simulink library "elementsLibrary"  (R2018a)
settings: Solver=VariableStepAuto  StartTime=0.0  StopTime=10.0  RelTol=1e-3
undefined symbols (not defined in the file): aerodynamics, ascent, avionics, environment, payload, propulsion, pvessel, recovery, rocket, sequencer
libraries: snippetLibrary x43, $bdroot x24, sharedutil x8, theirs_elementsLibrary x3, simulink_extras x1, aerolibutil x1
(part 2 of 4)

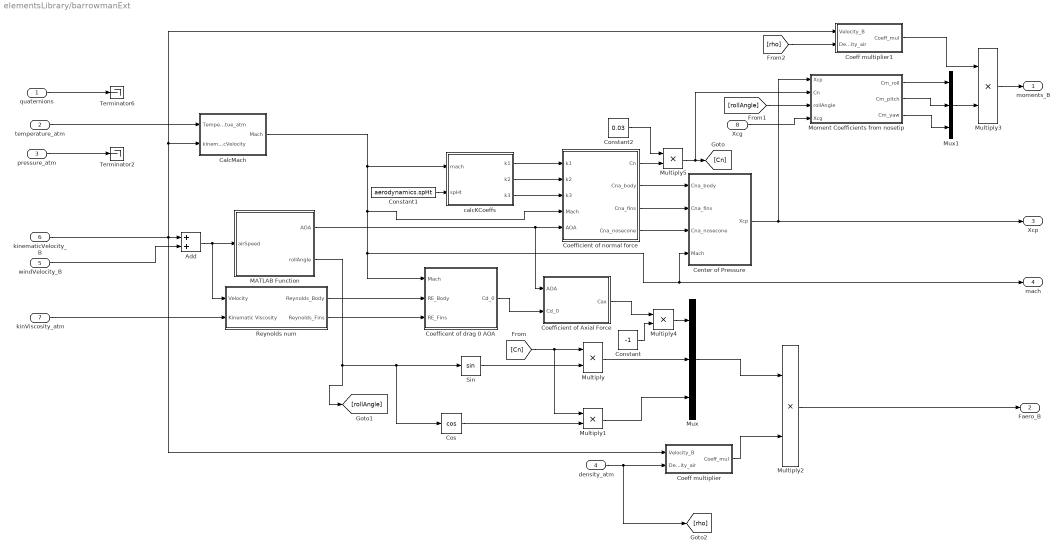
== system elementsLibrary/barrowmanExt ==
  quaternions : Inport
  temperature_atm : Inport  Port=2
  pressure_atm : Inport  Port=3
  density_atm : Inport  Port=4
  windVelocity_B : Inport  Port=5
  kinematicVelocity_B : Inport  Port=6
  kinViscosity_atm : Inport  Port=7
  Xcg : Inport  Port=8
  Add : Sum
  CalcMach : Subsystem
  Center of Pressure : Subsystem
  Coeff multiplier : Subsystem
  Coeff multiplier1 : Subsystem
  Coefficent of drag 0 AOA : Subsystem
  Coefficient of Axial Force : Subsystem
  Coefficient of normal force : Subsystem
  Constant : Constant  Value=-1
  Constant1 : Constant  Value=aerodynamics.spHt
  Constant2 : Constant  Value=0.03
  Cos : Trigonometry  Operator=cos
  MATLAB Function : MATLAB Function  TreatAsAtomicUnit=on
  Moment Coefficients from nosetip : Subsystem
  Multiply{,1..5} (6 alike) : Product
  Mux : Mux  Inputs=3
  Mux1 : Mux  Inputs=3
  Reynolds num : Subsystem
  Sin : Trigonometry
  Terminator2 : Terminator
  Terminator6 : Terminator
  calcKCoeffs : MATLAB Function  TreatAsAtomicUnit=on
  moments_B : Outport
  Faero_B : Outport  Port=2
  Xcp : Outport  Port=3
  mach : Outport  Port=4
  wires:
  pressure_atm/1 -> Terminator2/1
  temperature_atm/1 -> CalcMach/1(Temperatue_atm)
  kinViscosity_atm/1 -> Reynolds num/2(Kinematic Viscosity)
  quaternions/1 -> Terminator6/1
  Add/1 -> Reynolds num/1(Velocity), MATLAB Function/1(airSpeed)
  windVelocity_B/1 -> Add/2
  Reynolds num/1(Reynolds_Body) -> Coefficent of drag 0 AOA/2(RE_Body)
  Reynolds num/2(Reynolds_Fins) -> Coefficent of drag 0 AOA/3(RE_Fins)
  MATLAB Function/1(AOA) -> Coefficient of Axial Force/1(AOA), Coefficient of normal force/5(AOA)
  calcKCoeffs/3(k3) -> Coefficient of normal force/3(k3)
  calcKCoeffs/2(k2) -> Coefficient of normal force/2(k2)
  calcKCoeffs/1(k1) -> Coefficient of normal force/1(k1)
  Constant1/1 -> calcKCoeffs/2(spHt)
  Mux/1 -> Multiply2/1
  CalcMach/1(Mach) -> calcKCoeffs/1(mach), Coefficient of normal force/4(Mach), Coefficent of drag 0 AOA/1(Mach), Center of Pressure/4(Mach), mach/1
  Center of Pressure/1(Xcp) -> Xcp/1, Moment Coefficients from nosetip/1(Xcp)
  Coeff multiplier/1(Coeff_mul) -> Multiply2/2
  Coefficent of drag 0 AOA/1(Cd_0) -> Coefficient of Axial Force/2(Cd_0)
  Coefficient of normal force/2(Cna_body) -> Center of Pressure/1(Cna_body)
  Coefficient of normal force/3(Cna_fins) -> Center of Pressure/2(Cna_fins)
  Coefficient of normal force/4(Cna_nosecone) -> Center of Pressure/3(Cna_nosecone)
  [Cn] -> Multiply/1, Multiply1/1
  Multiply1/1 -> Mux/3
  Multiply2/1 -> Faero_B/1
  Multiply/1 -> Mux/2
  Sin/1 -> Multiply/2
  density_atm/1 -> [rho], Coeff multiplier/2(Density_air)
  kinematicVelocity_B/1 -> Coeff multiplier/1(Velocity_B), Add/1, CalcMach/2(kinematicVelocity), Coeff multiplier1/1(Velocity_B)
  Cos/1 -> Multiply1/2
  MATLAB Function/2(rollAngle) -> [rollAngle], Cos/1, Sin/1
  [rollAngle] -> Moment Coefficients from nosetip/3(rollAngle)
  Moment Coefficients from nosetip/1(Cm_roll) -> Mux1/1
  Moment Coefficients from nosetip/2(Cm_pitch) -> Mux1/2
  Moment Coefficients from nosetip/3(Cm_yaw) -> Mux1/3
  Mux1/1 -> Multiply3/2
  Coeff multiplier1/1(Coeff_mul) -> Multiply3/1
  Multiply3/1 -> moments_B/1
  [rho] -> Coeff multiplier1/2(Density_air)
  Xcg/1 -> Moment Coefficients from nosetip/4(Xcg)
  Multiply4/1 -> Mux/1
  Coefficient of Axial Force/1(Cax) -> Multiply4/1
  Constant/1 -> Multiply4/2
  Coefficient of normal force/1(Cn) -> Multiply5/2
  Multiply5/1 -> Moment Coefficients from nosetip/2(Cn), [Cn]
  Constant2/1 -> Multiply5/1

== system elementsLibrary/environment ==
  altitude_E : Inport
  Earthv1 : $bdroot/Earthv1  environment=environment
  windVelocity_E : Outport
  Temperature : Outport  Port=2
  Pressure : Outport  Port=3
  Density : Outport  Port=4
  kinViscosity_atm : Outport  Port=5
  constants : Outport  Port=6
  wires:
  altitude_E/1 -> Earthv1/1
  Earthv1/1 -> windVelocity_E/1
  Earthv1/2 -> Temperature/1
  Earthv1/3 -> Pressure/1
  Earthv1/4 -> Density/1
  Earthv1/5 -> kinViscosity_atm/1
  Earthv1/6 -> constants/1

== system elementsLibrary/nitrousTank1 ==
  massFlow : Inport
  temperature_atm : Inport  Port=2
  Add : Sum
  Enthalpy of Vapourization : Lookup_n-D  NumberOfTableDimensions=1  BreakpointsForDimension1=pvessel.temperatureBreakpoints  Table=pvessel.delHVap  InternalRulePriority=Speed  RndMeth=Simplest  InputSameDT=on
  Integrator : Integrator
  Integrator1 : Integrator  InitialCondition=pvessel.initOxiTemp
  Nitrous Liq Density : Lookup_n-D  NumberOfTableDimensions=1  BreakpointsForDimension1=pvessel.temperatureBreakpoints  Table=pvessel.liqDensity  InternalRulePriority=Speed  RndMeth=Simplest  InputSameDT=on
  Nitrous Vap Density : Lookup_n-D  NumberOfTableDimensions=1  BreakpointsForDimension1=pvessel.temperatureBreakpoints  Table=pvessel.vapDensity  InternalRulePriority=Speed  RndMeth=Simplest  InputSameDT=on
  Nitrous_Inertia_and_cg : Subsystem
  Saturation Pressures : Lookup_n-D  NumberOfTableDimensions=1  LookupTableObject=SatNitrousTable  BreakpointsForDimension1=pvessel.temperatureBreakpoints  Table=pvessel.pressure  InterpMethod=Linear Lagrange  ExtrapMethod=Clip  DiagnosticForOutOfRangeInput=Warning  InternalRulePriority=Speed  RndMeth=Simplest  InputSameDT=on
  Spec Heat Capacity : Lookup_n-D  NumberOfTableDimensions=1  BreakpointsForDimension1=pvessel.temperatureBreakpoints  Table=pvessel.specHeatCap  InternalRulePriority=Speed  RndMeth=Simplest  InputSameDT=on
  Terminator{,1..3} (4 alike) : Terminator
  Unit Delay : UnitDelay  InitialCondition=pvessel.initLiqMass  SampleTime=-1
  Unit Delay1 : UnitDelay  InitialCondition=pvessel.initOxiTemp  SampleTime=-1
  Unit Delay2 : UnitDelay  InitialCondition=0.001  SampleTime=-1
  Unit Delay3 : UnitDelay  InitialCondition=pvessel.initVapMass  SampleTime=-1
  Unit Delay4 : UnitDelay  InitialCondition=pvessel.initOxiTemp  SampleTime=-1
  Unit Delay5 : UnitDelay  InitialCondition=pvessel.initOxiTemp  SampleTime=-1
  nox_blowdown : MATLAB Function  TreatAsAtomicUnit=on  SystemSampleTime=timeStep  mask{timeStep=pvessel.timeStep, initOxiMass=pvessel.initOxiMass, initLiqMass=pvessel.initLiqMass, tankVolume=pvessel.volumeTank, n2o_pCrit=pvessel.n2o_pCrit, n2o_rhoCrit=pvessel.n2o_rhoCrit, n2o_tCrit=pvessel.n2o_tCrit, n2o_ZCrit=pvessel.n2o_ZCrit, n2o_gamma=pvessel.n2o_gamma}
  output_selection1 : MATLAB Function  TreatAsAtomicUnit=on
  sat_n20_temperature_calc : MATLAB Function  TreatAsAtomicUnit=on
  pressure : Outport
  mass : Outport  Port=2  PortDimensions=1
  rho_oxi : Outport  Port=3
  Oxi_inertia : Outport  Port=4
  X_cg_oxi_engine : Outport  Port=5
  wires:
  output_selection1/1(n2o_sel_p) -> pressure/1, Unit Delay4/1  "pNox"
  massFlow/1 -> Integrator/1
  temperature_atm/1 -> Terminator1/1
  Spec Heat Capacity/1 -> sat_n20_temperature_calc/2(specHtCp)  "specHCapNox"
  Enthalpy of Vapourization/1 -> sat_n20_temperature_calc/3(enthVap)  "enthVapNox"
  Nitrous Liq Density/1 -> output_selection1/4(satLiqDens), nox_blowdown/2(liquidDens)  "satRhoLiqNox"
  Nitrous Vap Density/1 -> nox_blowdown/3(vapDens)  "satRhoVapNox"
  Saturation Pressures/1 -> output_selection1/1(n2o_sat_pressure)
  nox_blowdown/2(liquidMass) -> Unit Delay/1  "liqMassNox"
  Integrator/1 -> nox_blowdown/1(massGone)
  nox_blowdown/4(vapourizedMass) -> Unit Delay2/1  "vapourizedMassNox"
  nox_blowdown/1(vapMass) -> Unit Delay3/1
  Unit Delay2/1 -> sat_n20_temperature_calc/5(vapourizedMass), nox_blowdown/6(oldVapourizedMass)
  Unit Delay/1 -> sat_n20_temperature_calc/4(liquidMass), nox_blowdown/5(oldLiquidMass), output_selection1/2(liquidMass), Add/2  "mass_oxi"
  sat_n20_temperature_calc/1(temperature) -> Unit Delay1/1
  sat_n20_temperature_calc/2(deltaTemp) -> Integrator1/1
  Unit Delay1/1 -> output_selection1/5(satLiqTemp), sat_n20_temperature_calc/1(oldTemperature), Spec Heat Capacity/1, Enthalpy of Vapourization/1, Nitrous Liq Density/1, Saturation Pressures/1, Nitrous Vap Density/1  "SatTemperatureNox"
  Integrator1/1 -> Terminator/1  "inte_delT"
  Unit Delay3/1 -> output_selection1/3(vapMass), Add/1  "vapMassNox"
  output_selection1/2(n2o_sel_rho) -> rho_oxi/1, Nitrous_Inertia_and_cg/2(density)  "rhoNox"
  nox_blowdown/5(vapourDens) -> output_selection1/6(vapDens)
  nox_blowdown/6(vapourTemp) -> output_selection1/7(vapTemp)
  output_selection1/3(n2o_sel_Temp) -> Terminator3/1, Unit Delay5/1  "tempNox"
  nox_blowdown/7(vapourPres) -> output_selection1/8(vapPres)
  Unit Delay4/1 -> nox_blowdown/4(tankPressure)
  Unit Delay5/1 -> nox_blowdown/7(vapTemp)
  Nitrous_Inertia_and_cg/1(Inertia_oxi) -> Oxi_inertia/1
  Nitrous_Inertia_and_cg/2(X_cg) -> X_cg_oxi_engine/1  "X_cg_oxi_engine"
  nox_blowdown/3(massProp) -> Terminator2/1
  Add/1 -> mass/1, Nitrous_Inertia_and_cg/1(mass)

== system elementsLibrary/payload ==
  In1 : Inport
  payload2021 : $bdroot/payload2021  payload=payload
  Out1 : Outport
  wires:
  In1/1 -> payload2021/1
  payload2021/1 -> Out1/1

== system elementsLibrary/payload2021 ==
  Env_temp : Inport
  Input : Inport  Port=2
  Input1 : Inport  Port=3
  Payload_Samples_Temperature : Outport
  Rate_of_Heat_Transfer_Env_Sample : Outport  Port=2
  Payload_Pressure : Outport  Port=3
  Total_Heat_Transfer : Outport  Port=4
  Mass_Dry_Ice : Outport  Port=5

== system elementsLibrary/propulsion ==
  time : Inport
  valveCmd : Inport  Port=2
  temp_atm : Inport  Port=3
  pressure_atm : Inport  Port=4
  "density_atm " : Inport  Port=5
  HREV1 : $bdroot/HREV1  propulsion=propulsion
  gnd{1..4} (4 alike) : Ground
  thrust_B : Outport
  Ve_gas : Outport  Port=2
  propellantMass : Outport  Port=3
  propellantInertias : Outport  Port=4
  engineProperties : Outport  Port=5
  Ve_gas1 : Outport  Port=6
  engineMass : Outport  Port=7
  wires:
  time/1 -> HREV1/1
  valveCmd/1 -> HREV1/2
  temp_atm/1 -> HREV1/3
  pressure_atm/1 -> HREV1/4
  "density_atm "/1 -> HREV1/5
  HREV1/1 -> thrust_B/1
  HREV1/4 -> propellantInertias/1
  HREV1/5 -> engineProperties/1
  HREV1/2 -> Ve_gas1/1
  HREV1/3 -> engineMass/1
  gnd2/1 -> Ve_gas/1
  gnd3/1 -> propellantMass/1

== system elementsLibrary/pvessel ==
  massFlow : Inport
  temperature_atm : Inport  Port=2
  nitrousTank1 : $bdroot/nitrousTank1  pvessel=pvessel
  pressure : Outport
  mass : Outport  Port=2
  rho_oxi : Outport  Port=3
  wires:
  massFlow/1 -> nitrousTank1/1
  temperature_atm/1 -> nitrousTank1/2
  nitrousTank1/1 -> pressure/1
  nitrousTank1/2 -> mass/1
  nitrousTank1/3 -> rho_oxi/1

== system elementsLibrary/recovery ==
  windVelocity : Inport
  density_atm : Inport  Port=2
  envConstants : Inport  Port=3
  inQuaternions : Inport  Port=4
  initVelocity_E : Inport  Port=5
  initPosition_E : Inport  Port=6
  inAngVel : Inport  Port=7
  descentOneDeploy : Inport  Port=8
  descentTwoDeploy : Inport  Port=9
  flightState : Inport  Port=10
  SingleChute : $bdroot/SingleChute  recovery=recovery
  orientationP : Outport
  angularVelocityP : Outport  Port=2
  angularAccelerationP : Outport  Port=3
  angularAccelerationR : Outport  Port=4
  orientationR : Outport  Port=5
  angularVelocityR : Outport  Port=6
  posP_E : Outport  Port=7
  posR_E : Outport  Port=8
  velocityP_E : Outport  Port=9
  velocityR_E : Outport  Port=10
  accelerationR_E : Outport  Port=11
  accelerationP_E : Outport  Port=12
  wires:
  windVelocity/1 -> SingleChute/1
  density_atm/1 -> SingleChute/2
  envConstants/1 -> SingleChute/3
  inQuaternions/1 -> SingleChute/4
  initVelocity_E/1 -> SingleChute/5
  initPosition_E/1 -> SingleChute/6
  inAngVel/1 -> SingleChute/7
  descentOneDeploy/1 -> SingleChute/8
  descentTwoDeploy/1 -> SingleChute/9
  flightState/1 -> SingleChute/10
  SingleChute/1 -> orientationP/1
  SingleChute/2 -> angularVelocityP/1
  SingleChute/3 -> angularAccelerationP/1
  SingleChute/4 -> angularAccelerationR/1
  SingleChute/5 -> orientationR/1
  SingleChute/6 -> angularVelocityR/1
  SingleChute/7 -> posP_E/1
  SingleChute/8 -> posR_E/1
  SingleChute/9 -> velocityP_E/1
  SingleChute/10 -> velocityR_E/1
  SingleChute/11 -> accelerationR_E/1
  SingleChute/12 -> accelerationP_E/1

== system elementsLibrary/rocket ==
  time : Inport
  Jackalope : $bdroot/Jackalope  rocket=rocket
  acceleration_E : Outport
  angularAcceleration_B : Outport  Port=2
  angularVelocity_B : Outport  Port=3
  position_E : Outport  Port=4
  orientation : Outport  Port=5
  velocity_E : Outport  Port=6
  wires:
  time/1 -> Jackalope/1
  Jackalope/1 -> acceleration_E/1
  Jackalope/2 -> angularAcceleration_B/1
  Jackalope/3 -> angularVelocity_B/1
  Jackalope/4 -> position_E/1
  Jackalope/5 -> orientation/1
  Jackalope/6 -> velocity_E/1

== system elementsLibrary/sequencer ==
  position_E : Inport
  orientation : Inport  Port=2
  velocity_E : Inport  Port=3
  thrust_B : Inport  Port=4
  descentOneDeploy : Inport  Port=5
  descentTwoDeploy : Inport  Port=6
  FSv1 : $bdroot/FSv1  sequencer=sequencer
  flightState : Outport
  towerVector : Outport  Port=2
  wires:
  position_E/1 -> FSv1/1
  orientation/1 -> FSv1/2
  velocity_E/1 -> FSv1/3
  thrust_B/1 -> FSv1/4
  descentOneDeploy/1 -> FSv1/5
  descentTwoDeploy/1 -> FSv1/6
  FSv1/1 -> flightState/1
  FSv1/2 -> towerVector/1

== system elementsLibrary/Ascentv1/Calculate Aero Coeffs & Center of Pressure ==
  kinematicVelocity_B : Inport
  temperpature_atm : Inport  Port=2
  pressure_atm : Inport  Port=3
  kinViscosity_atm : Inport  Port=4
  density_atm : Inport  Port=5
  windVelocity_B : Inport  Port=6
  Add1 : Sum
  Terminator{,1..6} (7 alike) : Terminator
  calcAeroCoeffs : MATLAB Function  TreatAsAtomicUnit=on  mask{lw=ascent.aerodynamics.lw, lr=ascent.aerodynamics.lr, lt=ascent.aerodynamics.lt, ls=ascent.aerodynamics.ls, A_fwt=ascent.aerodynamics.A_fwt, Ar=ascent.aerodynamics.Ar, Ap=ascent.aerodynamics.Ap, df=ascent.aerodynamics.df, nf=ascent.aerodynamics.nf, dn=ascent.aerodynamics.dn, du=ascent.aerodynamics.du, ln=ascent.aerodynamics.ln, lb=ascent.aerodynamics.lb, CNalpha_nose=ascent.aerodynamics.CNalpha_nose, Xcp_nose=ascent.aerodynamics.Xcp_nose, Xcp_body=ascent.aerodynamics.Xcp_body, Xcp_fins=ascent.aerodynamics.Xcp_fins, Xf=ascent.aerodynamics.Xf}
  calculate AOA & Side Slip : Subsystem
  calculate Mach : Subsystem
  calculate ZAOA_cd : Subsystem
  Ca_B : Outport
  Cy_B : Outport  Port=2
  Cz_B : Outport  Port=3
  Xcp : Outport  Port=4
  mach : Outport  Port=5
  wires:
  pressure_atm/1 -> Terminator1/1
  temperpature_atm/1 -> calculate Mach/1(temperature_atm)
  kinViscosity_atm/1 -> calculate ZAOA_cd/3(kinViscosity_atm)
  density_atm/1 -> calculate ZAOA_cd/2(density_atm)
  calculate Mach/2(speed of sound) -> Terminator2/1
  calculate Mach/1(mach) -> calcAeroCoeffs/1(mach), mach/1  "mach"
  Add1/1 -> calculate Mach/2(apparentVelocity_E), calculate AOA & Side Slip/1(apparentVelocity_B), calcAeroCoeffs/5(Va), calculate ZAOA_cd/1(apparentVelocity_B)  "Va_B"
  kinematicVelocity_B/1 -> Add1/1
  windVelocity_B/1 -> Add1/2
  calcAeroCoeffs/5(Xcp) -> Xcp/1  "Xcp"
  calcAeroCoeffs/4(Cz_B) -> Cz_B/1  "Cz_B"
  calcAeroCoeffs/3(Cy_B) -> Cy_B/1  "Cy_B"
  calcAeroCoeffs/2(Ca_B) -> Ca_B/1  "Ca_B"
  calcAeroCoeffs/1(Cn_B) -> Terminator/1  "Cn_B"
  calculate ZAOA_cd/1(ZAOA_cd) -> calcAeroCoeffs/2(cd)  "cd"
  calculate AOA & Side Slip/1(AOA) -> calcAeroCoeffs/3(AOA)  "AOA"
  calculate AOA & Side Slip/2(aeroRollAngle) -> calcAeroCoeffs/4(aeroRollAngle)  "aeroRollAngle"
  calcAeroCoeffs/6(Cm_B) -> Terminator3/1  "Cm_B"
  calcAeroCoeffs/7(CN_body) -> Terminator4/1  "CN_body"
  calcAeroCoeffs/8(CN_nose) -> Terminator5/1  "CN_nose"
  calcAeroCoeffs/9(CN_fins) -> Terminator6/1  "CN_fins"

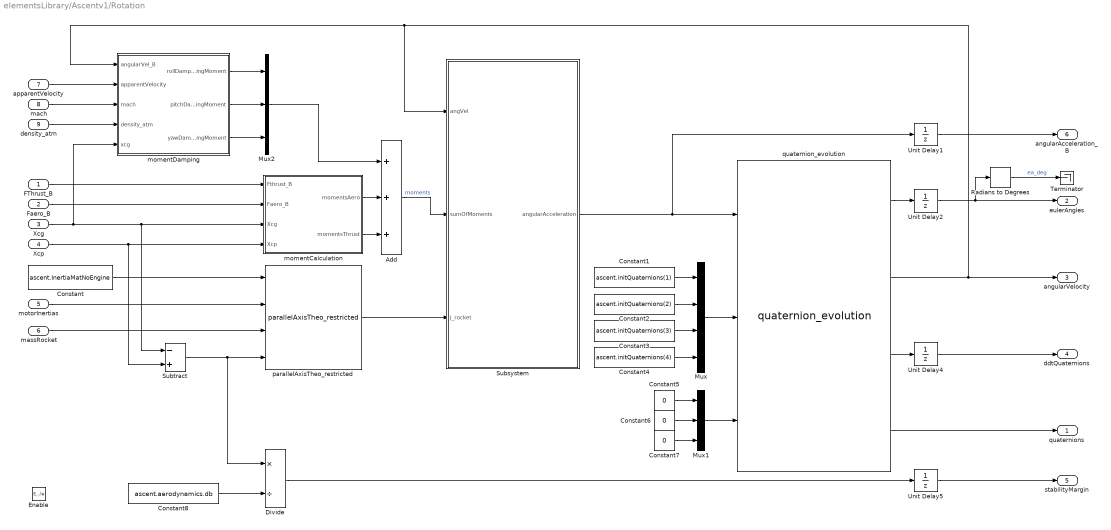
== system elementsLibrary/Ascentv1/Rotation ==
  FThrust_B : Inport
  Faero_B : Inport  Port=2
  Xcg : Inport  Port=3
  Xcp : Inport  Port=4
  motorInertias : Inport  Port=5
  massRocket : Inport  Port=6
  apparentVelocity : Inport  Port=7
  mach : Inport  Port=8
  density_atm : Inport  Port=9
  Enable : EnablePort  StatesWhenEnabling=reset
  Add : Sum  Inputs=3
  Constant : Constant  Value=ascent.InertiaMatNoEngine
  Constant1 : Constant  Value=ascent.initQuaternions(1)
  Constant2 : Constant  Value=ascent.initQuaternions(2)
  Constant3 : Constant  Value=ascent.initQuaternions(3)
  Constant4 : Constant  Value=ascent.initQuaternions(4)
  Constant5 : Constant  Value=0
  Constant6 : Constant  Value=0
  Constant7 : Constant  Value=0
  Constant8 : Constant  Value=ascent.aerodynamics.db
  Divide : Product  Inputs=*/
  Mux : Mux
  Mux1 : Mux  Inputs=3
  Mux2 : Mux  Inputs=3
  Radians to Degrees : simulink_extras/Transformations/Radians to Degrees
  Subsystem : Subsystem
  Subtract : Sum  Inputs=-+
  Terminator : Terminator
  Unit Delay{1..2,4..5} (4 alike) : UnitDelay  SampleTime=-1
  momentCalculation : Subsystem
  momentDamping : Subsystem
  parallelAxisTheo_restricted : snippetLibrary/dynamicsSnippets/parallelAxisTheo_restricted
  quaternion_evolution : snippetLibrary/mathSnippets/quaternion_evolution
  quaternions : Outport
  eulerAngles : Outport  Port=2
  angularVelocity : Outport  Port=3
  ddtQuaternions : Outport  Port=4
  stabilityMargin : Outport  Port=5
  angularAcceleration_B : Outport  Port=6
  wires:
  quaternion_evolution/1 -> Unit Delay2/1
  FThrust_B/1 -> momentCalculation/1(Fthrust_B)
  Faero_B/1 -> momentCalculation/2(Faero_B)
  motorInertias/1 -> parallelAxisTheo_restricted/2
  Constant/1 -> parallelAxisTheo_restricted/1
  massRocket/1 -> parallelAxisTheo_restricted/3
  parallelAxisTheo_restricted/1 -> Subsystem/3(J_rocket)
  quaternion_evolution/3 -> Unit Delay4/1
  Mux/1 -> quaternion_evolution/2
  Constant1/1 -> Mux/1
  Constant2/1 -> Mux/2
  Constant3/1 -> Mux/3
  Constant4/1 -> Mux/4
  Subtract/1 -> parallelAxisTheo_restricted/4, Divide/1
  Xcp/1 -> momentCalculation/4(Xcp), Subtract/2
  Xcg/1 -> momentDamping/5(xcg), momentCalculation/3(Xcg), Subtract/1
  Mux1/1 -> quaternion_evolution/3
  Constant5/1 -> Mux1/1
  Constant6/1 -> Mux1/2
  Constant7/1 -> Mux1/3
  Subsystem/1(angularAcceleration) -> Unit Delay1/1, quaternion_evolution/1
  quaternion_evolution/4 -> quaternions/1
  Unit Delay2/1 -> Radians to Degrees/1, eulerAngles/1
  quaternion_evolution/2 -> angularVelocity/1, Subsystem/1(angVel), momentDamping/1(angularVel_B)
  Unit Delay4/1 -> ddtQuaternions/1
  Unit Delay5/1 -> stabilityMargin/1
  Unit Delay1/1 -> angularAcceleration_B/1
  Radians to Degrees/1 -> Terminator/1  "ea_deg"
  Divide/1 -> Unit Delay5/1
  Constant8/1 -> Divide/2
  mach/1 -> momentDamping/3(mach)
  apparentVelocity/1 -> momentDamping/2(apparentVelocity)
  momentDamping/1(rollDampingMoment) -> Mux2/1
  momentDamping/2(pitchDampingMoment) -> Mux2/2
  momentDamping/3(yawDampingMoment) -> Mux2/3
  Mux2/1 -> Add/1
  momentCalculation/1(momentsAero) -> Add/2
  momentCalculation/2(momentsThrust) -> Add/3
  Add/1 -> Subsystem/2(sumOfMoments)  "moments"
  density_atm/1 -> momentDamping/4(density_atm)

== system elementsLibrary/Ascentv1/Tower_Correction ==
  flightState : Inport
  quaternionsIn : Inport  Port=2
  eulerAnglesIn : Inport  Port=3
  angularVelocityIn : Inport  Port=4
  ddtQuaternionsIn : Inport  Port=5
  stabilityMarginIn : Inport  Port=6
  angularAccelerationIn_B : Inport  Port=7
  Constant : Constant
  Constant1 : Constant  Value=ascent.initQuaternions(1)
  Constant{5..11} (7 alike) : Constant  Value=0
  Constant2 : Constant  Value=ascent.initQuaternions(2)
  Constant3 : Constant  Value=ascent.initQuaternions(3)
  Constant4 : Constant  Value=ascent.initQuaternions(4)
  Mux : Mux
  Mux1 : Mux  Inputs=3
  Mux2 : Mux
  NotEqual : RelationalOperator  Operator=~=  OutDataTypeStr=boolean  RndMeth=Simplest
  Switch{,2..3,5} (4 alike) : Switch  Criteria=u2 ~= 0
  quaternions : Outport
  eulerAngles : Outport  Port=2
  angularVelocity : Outport  Port=3
  ddtQuaternions : Outport  Port=4
  stabilityMargin : Outport  Port=5
  angularAcceleration_B : Outport  Port=6
  wires:
  quaternionsIn/1 -> Switch/1
  Switch/1 -> quaternions/1
  angularVelocityIn/1 -> Switch2/1
  ddtQuaternionsIn/1 -> Switch3/1
  angularAccelerationIn_B/1 -> Switch5/1
  eulerAnglesIn/1 -> eulerAngles/1
  Switch2/1 -> angularVelocity/1
  Switch3/1 -> ddtQuaternions/1
  stabilityMarginIn/1 -> stabilityMargin/1
  Switch5/1 -> angularAcceleration_B/1
  flightState/1 -> NotEqual/1
  Constant/1 -> NotEqual/2
  NotEqual/1 -> Switch3/2, Switch5/2, Switch2/2, Switch/2
  Constant1/1 -> Mux/1
  Constant2/1 -> Mux/2
  Constant3/1 -> Mux/3
  Constant5/1 -> Mux1/1
  Constant6/1 -> Mux1/2
  Mux/1 -> Switch/3
  Constant7/1 -> Mux1/3
  Constant4/1 -> Mux/4
  Mux1/1 -> Switch2/3, Switch5/3
  Constant10/1 -> Mux2/3
  Constant8/1 -> Mux2/1
  Constant9/1 -> Mux2/2
  Mux2/1 -> Switch3/3
  Constant11/1 -> Mux2/4

== system elementsLibrary/Ascentv1/Translation ==
  Faero_E : Inport
  FThrust_E : Inport  Port=2
  Fg_E : Inport  Port=3
  massRocket : Inport  Port=4
  Enable : EnablePort  StatesWhenEnabling=reset
  Add : Sum  Inputs=+++
  Divide : Product  Inputs=*/
  Integrator : Integrator
  Integrator1 : Integrator  InitialCondition=[0;0;ascent.aerodynamics.l_TR/2]
  position_E : Outport
  velocity_E : Outport  Port=2
  acceleration_E : Outport  Port=3
  wires:
  Fg_E/1 -> Add/3
  Faero_E/1 -> Add/1
  FThrust_E/1 -> Add/2
  Add/1 -> Divide/1
  massRocket/1 -> Divide/2
  Divide/1 -> acceleration_E/1, Integrator/1  "acceleration_E"
  Integrator/1 -> velocity_E/1, Integrator1/1  "velocity_E"
  Integrator1/1 -> position_E/1  "position_E"

== system elementsLibrary/Ascentv1/center of mass//gravity calculation ==
  motorMass : Inport
  motorProperties : Inport  Port=2
  rocketEmptyMass : Inport  Port=3
  rocketEmptyXcg : Inport  Port=4
  Add : Sum
  Add1 : Sum
  Add2 : Sum
  Bus Selector : BusSelector  OutputSignals=x_gm_B,x_cg_B
  Divide : Product  Inputs=*/
  Multiply : Product
  Multiply1 : Product
  Xcg : Outport
  massR : Outport  Port=2
  wires:
  motorProperties/1 -> Bus Selector/1
  Bus Selector/2 -> Add/2  "<x_cg_B>"
  Bus Selector/1 -> Add/1  "<x_gm_B>"
  motorMass/1 -> Multiply/1, Add2/1
  Add/1 -> Multiply/2
  Multiply/1 -> Add1/2
  rocketEmptyMass/1 -> Multiply1/2, Add2/2
  rocketEmptyXcg/1 -> Multiply1/1
  Divide/1 -> Xcg/1
  Add2/1 -> massR/1, Divide/2
  Add1/1 -> Divide/1
  Multiply1/1 -> Add1/1

== system elementsLibrary/Ascentv2/Calculating Mass and XCG ==
  rocketEmptyXcg : Inport
  rocketEmptyMass : Inport  Port=2
  propellantMass : Inport  Port=3
  motorProperties : Inport  Port=4
  Add : Sum
  Add1 : Sum
  Add2 : Sum
  Bus Selector : BusSelector  OutputSignals=x_gm_B,x_cg_B
  Divide : Product  Inputs=*/
  Multiply : Product
  Multiply1 : Product
  massRocket : Outport
  Xcg : Outport  Port=2
  wires:
  Bus Selector/2 -> Add/2  "<x_cg_B>"
  Add2/1 -> massRocket/1, Divide/2
  Divide/1 -> Xcg/1
  rocketEmptyMass/1 -> Multiply1/2, Add2/1
  Add/1 -> Multiply/2
  propellantMass/1 -> Add2/2, Multiply/1
  Bus Selector/1 -> Add/1  "<x_gm_B>"
  Multiply1/1 -> Add1/1
  Add1/1 -> Divide/1
  Multiply/1 -> Add1/2
  rocketEmptyXcg/1 -> Multiply1/1
  motorProperties/1 -> Bus Selector/1

== system elementsLibrary/Ascentv2/Force of Gravity ==
  G_Const : Inport
  massEarth : Inport  Port=2
  radiusEarth : Inport  Port=3
  massRocket : Inport  Port=4
  Altitude : Inport  Port=5
  Add : Sum
  Divide : Product  Inputs=*/
  Gain : Gain  Gain=-1
  Multiply : Product  Inputs=3
  Square : Math  Operator=square  SaturateOnIntegerOverflow=on
  Fg_E : Outport
  wires:
  massRocket/1 -> Multiply/3
  radiusEarth/1 -> Add/1
  Divide/1 -> Fg_E/1
  Altitude/1 -> Add/2
  Add/1 -> Square/1
  Square/1 -> Divide/2
  G_Const/1 -> Multiply/1
  massEarth/1 -> Multiply/2
  Multiply/1 -> Gain/1
  Gain/1 -> Divide/1

== system elementsLibrary/Ascentv2/Forces Body Frame to Earth Frame ==
  Transformation_Matrix : Inport
  F_Aero_B : Inport  Port=2
  F_Thrust_B : Inport  Port=3
  Matrix Multiply : Product  Multiplication=Matrix(*)
  Matrix Multiply1 : Product  Multiplication=Matrix(*)
  F_Aero_E : Outport
  F_Thrust_E : Outport  Port=2
  wires:
  Transformation_Matrix/1 -> Matrix Multiply1/1, Matrix Multiply/1
  F_Aero_B/1 -> Matrix Multiply1/2
  F_Thrust_B/1 -> Matrix Multiply/2
  Matrix Multiply1/1 -> F_Aero_E/1
  Matrix Multiply/1 -> F_Thrust_E/1

== system elementsLibrary/Ascentv2/Rotational ==
  moments_B : Inport
  propellentInertias : Inport  Port=2
  propellantMass : Inport  Port=3
  motorProperties : Inport  Port=4
  rocketEmptyXcg : Inport  Port=5
  Constant1 : Constant  Value=ascent.initQuaternions(1)
  Constant2 : Constant  Value=ascent.initQuaternions(2)
  Constant3 : Constant  Value=ascent.initQuaternions(3)
  Constant4 : Constant  Value=ascent.initQuaternions(4)
  Constant5 : Constant  Value=0.000001
  Constant6 : Constant  Value=0.000001
  Constant7 : Constant  Value=0.000001
  "Inertia_Matrix " : Subsystem
  Mux : Mux
  Mux1 : Mux  Inputs=3
  Subsystem : Subsystem
  Unit Delay{,1..3} (4 alike) : UnitDelay  SampleTime=-1
  quaternion_evolution : Subsystem
  quaternions : Outport
  ddtQuaternions : Outport  Port=2
  eulerAngles : Outport  Port=3
  angularVelocity : Outport  Port=4
  angularAcceleration_B : Outport  Port=5
  wires:
  quaternion_evolution/2(anguarVelocity) -> Unit Delay3/1, angularVelocity/1
  quaternion_evolution/4(quaternions) -> quaternions/1
  Mux/1 -> quaternion_evolution/2(initialQuaternions)
  Constant2/1 -> Mux/2
  Constant5/1 -> Mux1/1
  Constant3/1 -> Mux/3
  Constant6/1 -> Mux1/2
  Constant1/1 -> Mux/1
  Constant7/1 -> Mux1/3
  Constant4/1 -> Mux/4
  Mux1/1 -> quaternion_evolution/3(initialAngVel)
  moments_B/1 -> Subsystem/3(sumOfMoments)
  "Inertia_Matrix "/1(J_rocket) -> Subsystem/2(J_rocket)  "J equivelant"
  propellentInertias/1 -> "Inertia_Matrix "/1(motorInertias)
  propellantMass/1 -> "Inertia_Matrix "/2(propellantMass)
  motorProperties/1 -> "Inertia_Matrix "/3(motorProperties)
  rocketEmptyXcg/1 -> "Inertia_Matrix "/4(rocketEmptyXcg)
  quaternion_evolution/3(ddtQuaternions) -> Unit Delay/1
  Unit Delay/1 -> ddtQuaternions/1
  Unit Delay1/1 -> eulerAngles/1
  quaternion_evolution/1(euler_angles) -> Unit Delay1/1
  Subsystem/1(angularAcceleration) -> Unit Delay2/1
  Unit Delay2/1 -> angularAcceleration_B/1, quaternion_evolution/1(angularAccelerations_B)
  Unit Delay3/1 -> Subsystem/1(angVel)

== system elementsLibrary/Ascentv2/Tower_Correction ==
  flightState : Inport
  quaternionsIn : Inport  Port=2
  ddtQuaternionsIn : Inport  Port=3
  eulerAnglesIn : Inport  Port=4
  angularVelocityIn : Inport  Port=5
  stabilityMarginIn : Inport  Port=6
  angularAccelerationIn_B : Inport  Port=7
  Constant : Constant
  Constant1 : Constant  Value=ascent.initQuaternions(1)
  Constant{5..11} (7 alike) : Constant  Value=0
  Constant2 : Constant  Value=ascent.initQuaternions(2)
  Constant3 : Constant  Value=ascent.initQuaternions(3)
  Constant4 : Constant  Value=ascent.initQuaternions(4)
  Mux : Mux
  Mux1 : Mux  Inputs=3
  Mux2 : Mux
  NotEqual : RelationalOperator  Operator=~=  OutDataTypeStr=boolean  RndMeth=Simplest
  Switch{,2..3,5} (4 alike) : Switch  Criteria=u2 ~= 0
  quaternions : Outport
  eulerAngles : Outport  Port=2
  angularVelocity : Outport  Port=3
  ddtQuaternions : Outport  Port=4
  stabilityMargin : Outport  Port=5
  angularAcceleration_B : Outport  Port=6
  wires:
  quaternionsIn/1 -> Switch/1
  Switch/1 -> quaternions/1
  angularVelocityIn/1 -> Switch2/1
  ddtQuaternionsIn/1 -> Switch3/1
  angularAccelerationIn_B/1 -> Switch5/1
  eulerAnglesIn/1 -> eulerAngles/1
  Switch2/1 -> angularVelocity/1
  Switch3/1 -> ddtQuaternions/1
  stabilityMarginIn/1 -> stabilityMargin/1
  Switch5/1 -> angularAcceleration_B/1
  flightState/1 -> NotEqual/1
  Constant/1 -> NotEqual/2
  NotEqual/1 -> Switch3/2, Switch5/2, Switch2/2, Switch/2
  Constant1/1 -> Mux/1
  Constant2/1 -> Mux/2
  Constant3/1 -> Mux/3
  Constant5/1 -> Mux1/1
  Constant6/1 -> Mux1/2
  Mux/1 -> Switch/3
  Constant7/1 -> Mux1/3
  Constant4/1 -> Mux/4
  Mux1/1 -> Switch2/3, Switch5/3
  Constant10/1 -> Mux2/3
  Constant8/1 -> Mux2/1
  Constant9/1 -> Mux2/2
  Mux2/1 -> Switch3/3
  Constant11/1 -> Mux2/4

== system elementsLibrary/Ascentv2/Translational  ==
  F_Aero_E : Inport
  F_Thrust_E : Inport  Port=2
  Fg_E : Inport  Port=3
  massRocket : Inport  Port=4
  Add : Sum  Inputs=+++
  Divide : Product  Inputs=*/
  Integrator : Integrator
  Integrator1 : Integrator
  Acceleration_E : Outport
  Velocity_E : Outport  Port=2
  Position_E : Outport  Port=3
  wires:
  Integrator1/1 -> Position_E/1
  Divide/1 -> Integrator/1, Acceleration_E/1
  F_Aero_E/1 -> Add/1
  massRocket/1 -> Divide/2
  Integrator/1 -> Velocity_E/1, Integrator1/1
  F_Thrust_E/1 -> Add/2
  Fg_E/1 -> Add/3
  Add/1 -> Divide/1

== system elementsLibrary/Ascentv2/aerodynamics ==
  quaternions : Inport
  airbrakecmd : Inport  Port=2
  temperature_atm : Inport  Port=3
  pressure_atm : Inport  Port=4
  density_atm : Inport  Port=5
  windVelocity_E : Inport  Port=6
  kinematicVelocity_E : Inport  Port=7
  kinViscosity_atm : Inport  Port=8
  Xcg : Inport  Port=9
  Transformation_Matrix : Inport  Port=10
  Invert 3x3 Matrix : aerolibutil/Invert  3x3 Matrix
  Matrix Multiply : Product  Multiplication=Matrix(*)
  Matrix Multiply1 : Product  Multiplication=Matrix(*)
  Terminator1 : Terminator
  barrowmanExt : $bdroot/barrowmanExt  aerodynamics=aerodynamics
  moments_B : Outport
  Faero_B : Outport  Port=2
  Xcp : Outport  Port=3
  mach : Outport  Port=4
  wires:
  barrowmanExt/2 -> Faero_B/1
  pressure_atm/1 -> barrowmanExt/3
  airbrakecmd/1 -> Terminator1/1
  windVelocity_E/1 -> Matrix Multiply/2
  kinematicVelocity_E/1 -> Matrix Multiply1/2
  kinViscosity_atm/1 -> barrowmanExt/7
  density_atm/1 -> barrowmanExt/4
  temperature_atm/1 -> barrowmanExt/2
  quaternions/1 -> barrowmanExt/1
  barrowmanExt/1 -> moments_B/1
  barrowmanExt/3 -> Xcp/1
  barrowmanExt/4 -> mach/1
  Xcg/1 -> barrowmanExt/8
  Transformation_Matrix/1 -> Invert 3x3 Matrix/1
  Invert 3x3 Matrix/1 -> Matrix Multiply1/1, Matrix Multiply/1
  Matrix Multiply1/1 -> barrowmanExt/6
  Matrix Multiply/1 -> barrowmanExt/5

== system elementsLibrary/Earthv1/Wind Velocity Calculation ==
  In1 : Inport
  Altitude : Inport  Port=2
  Atmospheric coefficient : Constant  Value=environment.atmospheric_coeff
  Divide : Product  Inputs=*/
  Height at ground : Constant  Value=environment.referenceWindAltitude
  Multiply : Product
  Power : Math  Operator=pow  SaturateOnIntegerOverflow=on
  Wind Velocity at Ground : Constant  Value=environment.referenceWindSpeed
  Out1 : Outport
  wires:
  Height at ground/1 -> Divide/2
  In1/1 -> Divide/1
  Divide/1 -> Power/1
  Power/1 -> Multiply/1
  Wind Velocity at Ground/1 -> Multiply/2
  Atmospheric coefficient/1 -> Power/2
  Multiply/1 -> Out1/1

== system elementsLibrary/Earthv2/Gravitational Acceleration ==
  Altitude : Inport
  Earth Radius : Inport  Port=2
  Add : Sum
  Constant1 : Constant  Value=environment.MASS_EARTH
  Constant3 : Constant  Value=environment.GRAVITATION_CONST
  Divide : Product  Inputs=*/
  Gain : Gain  Gain=-1
  Multiply : Product
  Square : Math  Operator=square  SaturateOnIntegerOverflow=on
  Acceleration : Outport
  wires:
  Gain/1 -> Acceleration/1
  Divide/1 -> Gain/1
  Multiply/1 -> Divide/1
  Constant3/1 -> Multiply/2
  Constant1/1 -> Multiply/1
  Square/1 -> Divide/2
  Add/1 -> Square/1
  Earth Radius/1 -> Add/2
  Altitude/1 -> Add/1

== system elementsLibrary/Earthv2/Subsystem ==
  Latitude : Inport
  Add : Sum
  Cos1 : Trigonometry  Operator=cos
  Major Radius : Constant  Value=environment.MAJOR_RADIUS_EARTH
  Minor Radius : Constant  Value=environment.MINOR_RADIUS_EARTH
  Multiply2 : Product
  Multiply3 : Product
  Sin1 : Trigonometry
  Sqrt : Sqrt  SaturateOnIntegerOverflow=on
  Square : Math  Operator=square  SaturateOnIntegerOverflow=on
  Square1 : Math  Operator=square  SaturateOnIntegerOverflow=on
  Radius : Outport
  wires:
  Sqrt/1 -> Radius/1
  Minor Radius/1 -> Multiply2/1
  Sin1/1 -> Multiply3/2
  Major Radius/1 -> Multiply3/1
  Multiply2/1 -> Square/1
  Add/1 -> Sqrt/1
  Multiply3/1 -> Square1/1
  Cos1/1 -> Multiply2/2
  Square1/1 -> Add/2
  Square/1 -> Add/1
  Latitude/1 -> Cos1/1, Sin1/1

== system elementsLibrary/Earthv2/Wind Velocity Calculation ==
  Altitude : Inport
  Ground Wind Speed : Inport  Port=2
  Atmospheric coefficient : Constant  Value=environment.atmospheric_coeff
  Divide : Product  Inputs=*/
  Height at ground : Constant  Value=environment.referenceWindAltitude
  Multiply : Product
  Power : Math  Operator=pow  SaturateOnIntegerOverflow=on
  Out1 : Outport
  wires:
  Ground Wind Speed/1 -> Multiply/2
  Multiply/1 -> Out1/1
  Atmospheric coefficient/1 -> Power/2
  Power/1 -> Multiply/1
  Divide/1 -> Power/1
  Altitude/1 -> Divide/1
  Height at ground/1 -> Divide/2

== system elementsLibrary/HREV1/Chamber_Ballistics ==
  mdot_oxi : Inport
  cStar : Inport  Port=2
  Add : Sum
  Constant : Constant  Value=2
  Divide : Product  Inputs=*/
  Grain_outer_dia : Constant  Value=propulsion.Dfg_outer
  Inertia : Subsystem
  Integrator : Integrator  InitialCondition=propulsion.Dfg_inner
  Unit Delay : UnitDelay  SampleTime=-1
  X_grain_length : Constant  Value=propulsion.Lfg
  calc_chamber_params : Subsystem
  calc_mdot_fuel : Subsystem
  calc_port_diameter : Subsystem
  mdot_fuel : Outport
  mdot_total : Outport  Port=2
  Pc : Outport  Port=3
  Tc : Outport  Port=4
  rdot_fuel : Outport  Port=5
  massFlux_oxi : Outport  Port=6
  OF_ratio : Outport  Port=7
  mass_fuel : Outport  Port=8
  Fuel_inertia : Outport  Port=9
  X_cg_fuel : Outport  Port=10
  wires:
  mdot_oxi/1 -> Add/2, calc_port_diameter/1(mdot_oxi), calc_mdot_fuel/1(mdot_oxi)
  calc_port_diameter/1(dDp_dt) -> Integrator/1
  Integrator/1 -> calc_port_diameter/2(Dp_prev), calc_mdot_fuel/2(Dp), Inertia/2(Grain_inner_dia)  "D_port"
  calc_mdot_fuel/1(Gox) -> massFlux_oxi/1
  Add/1 -> mdot_total/1, calc_chamber_params/2(mdot_prop)
  calc_mdot_fuel/3(mdot_f) -> Add/1, mdot_fuel/1
  calc_mdot_fuel/2(rdot_f) -> Unit Delay/1, rdot_fuel/1
  calc_mdot_fuel/4(OF_ratio) -> calc_chamber_params/1(OF_ratio), OF_ratio/1
  calc_chamber_params/2(Tc) -> Tc/1
  calc_chamber_params/1(Pc) -> Pc/1
  cStar/1 -> calc_chamber_params/3(cStar)
  Unit Delay/1 -> calc_port_diameter/3(rdot_f)
  calc_mdot_fuel/5(massFuel) -> mass_fuel/1, Inertia/1(massFuel)
  Grain_outer_dia/1 -> Inertia/3(Grain_outer_dia)
  X_grain_length/1 -> Divide/1, Inertia/4(X_fuel_length)
  Inertia/1(Fuel_inertia) -> Fuel_inertia/1
  Constant/1 -> Divide/2
  Divide/1 -> X_cg_fuel/1

== system elementsLibrary/HREV1/Injecter ==
  "Tank_pressure " : Inport
  Chamber_pressure : Inport  Port=2
  density_oxi : Inport  Port=3
  mass_oxi : Inport  Port=4
  Area_of_injector_hole : Constant  Value=propulsion.A_ih
  Constant : Constant  Value=2
  Constant1 : Constant  Value=0
  GreaterThan : RelationalOperator  Operator=>  OutDataTypeStr=boolean  RndMeth=Simplest
  Injector_discharge_coefficient : Constant  Value=propulsion.injector_Cd
  Kpa_to_Pa : Gain  Gain=1000
  Less Than : RelationalOperator  OutDataTypeStr=boolean  RndMeth=Simplest
  Multiply : Product  Inputs=3
  Multiply1 : Product  Inputs=3
  Multiply2 : Product
  Multiply3 : Product
  Number_of_injector_holes : Constant  Value=propulsion.nIHoles
  Product : Product
  Saturation : Saturate  UpperLimit=10  LowerLimit=0
  Sqrt : Sqrt  SaturateOnIntegerOverflow=on
  Subtract : Sum  Inputs=+-
  mdot_oxi : Outport
  wires:
  Sqrt/1 -> Product/2
  density_oxi/1 -> Multiply1/2
  Constant/1 -> Multiply1/1
  Multiply/1 -> Product/1
  "Tank_pressure "/1 -> Less Than/1, Subtract/1
  Multiply1/1 -> Multiply2/1
  Area_of_injector_hole/1 -> Multiply/2
  Number_of_injector_holes/1 -> Multiply/3
  Product/1 -> Multiply3/1
  Injector_discharge_coefficient/1 -> Multiply/1
  Chamber_pressure/1 -> Less Than/2, Subtract/2
  Subtract/1 -> Kpa_to_Pa/1
  Saturation/1 -> mdot_oxi/1
  Kpa_to_Pa/1 -> Multiply1/3
  Less Than/1 -> Multiply2/2
  Multiply2/1 -> Sqrt/1
  mass_oxi/1 -> GreaterThan/1
  Constant1/1 -> GreaterThan/2
  GreaterThan/1 -> Multiply3/2
  Multiply3/1 -> Saturation/1

== system elementsLibrary/HREV1/Nozzle ==
  mdot : Inport
  Pc : Inport  Port=2
  Tc : Inport  Port=3
  P_atm : Inport  Port=4
  Constant : Constant  Value=0
  Divide : Product  Inputs=*/
  Mux : Mux  Inputs=3
  calc_Vexit : Subsystem
  calc_charVel : Subsystem
  calc_speedOfSound : Subsystem
  calc_thrust : Subsystem
  thrust_B : Outport
  V_exit : Outport  Port=2
  mach_exit : Outport  Port=3
  charV : Outport  Port=4
  wires:
  calc_charVel/1(cStar) -> charV/1
  calc_speedOfSound/1("speedOfSound ") -> Divide/2, calc_charVel/1(speedOfSound)
  Tc/1 -> calc_speedOfSound/1(Tc), calc_Vexit/1(Tc)
  calc_Vexit/1(Ve_gas) -> calc_thrust/2(Ve_gas), Divide/1, V_exit/1
  Divide/1 -> mach_exit/1
  Mux/1 -> thrust_B/1
  Constant/1 -> Mux/2, Mux/3
  P_atm/1 -> calc_thrust/4(Patm), calc_thrust/3(Pe), calc_Vexit/3(Pe)
  Pc/1 -> calc_Vexit/2(Pc)
  calc_thrust/1(axialThrust) -> Mux/1
  mdot/1 -> calc_thrust/1(mdot_prop)

== system elementsLibrary/HREV1/Propellant_Mass ==
  mass_oxi : Inport
  mass_fuel : Inport  Port=2
  Add1 : Sum
  massProp : Outport
  wires:
  Add1/1 -> massProp/1
  mass_oxi/1 -> Add1/1
  mass_fuel/1 -> Add1/2

== system elementsLibrary/HREV1/cg_propellent_engine ==
  X_cg_fuel_engine : Inport
  mass_fuel : Inport  Port=2
  X_cg_oxi_engine : Inport  Port=3
  mass_oxi : Inport  Port=4
  Add : Sum
  Add1 : Sum
  Divide : Product  Inputs=*/
  Multiply : Product
  Multiply1 : Product
  cg_prop_engine : Outport
  wires:
  mass_fuel/1 -> Add1/1, Multiply/2
  X_cg_fuel_engine/1 -> Multiply/1
  X_cg_oxi_engine/1 -> Multiply1/1
  mass_oxi/1 -> Add1/2, Multiply1/2
  Multiply/1 -> Add/1
  Multiply1/1 -> Add/2
  Add/1 -> Divide/1
  Add1/1 -> Divide/2
  Divide/1 -> cg_prop_engine/1

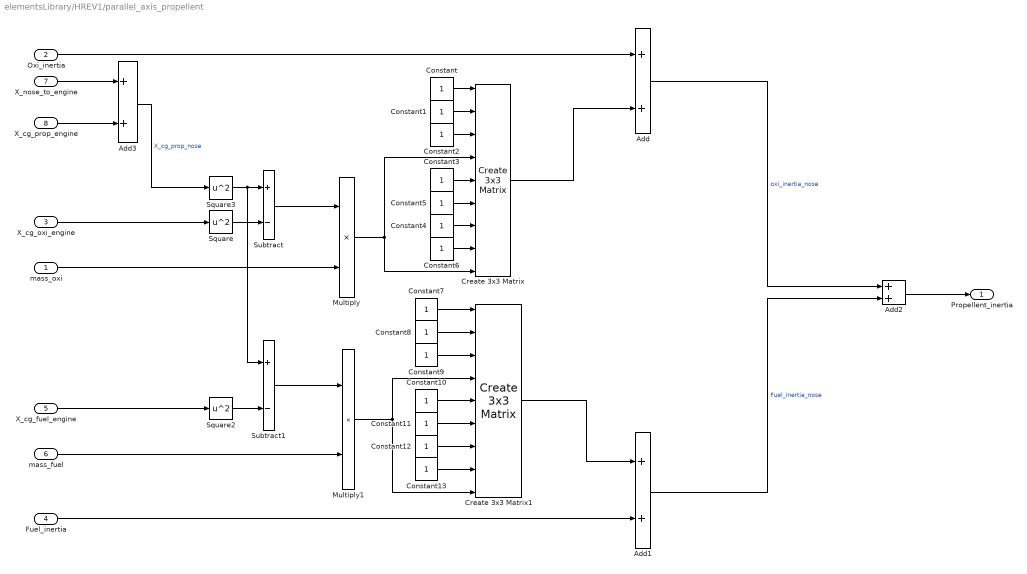
== system elementsLibrary/HREV1/parallel_axis_propellent ==
  mass_oxi : Inport
  Oxi_inertia : Inport  Port=2
  X_cg_oxi_engine : Inport  Port=3
  Fuel_inertia : Inport  Port=4
  X_cg_fuel_engine : Inport  Port=5
  mass_fuel : Inport  Port=6
  X_nose_to_engine : Inport  Port=7
  X_cg_prop_engine : Inport  Port=8
  Add{,1..3} (4 alike) : Sum
  Constant{,1..13} (14 alike) : Constant
  Create 3x3 Matrix : sharedutil/Create 3x3 Matrix  aMode=aMode
  Create 3x3 Matrix1 : sharedutil/Create 3x3 Matrix  aMode=aMode
  Multiply : Product
  Multiply1 : Product
  Square : Math  Operator=square  SaturateOnIntegerOverflow=on
  Square2 : Math  Operator=square  SaturateOnIntegerOverflow=on
  Square3 : Math  Operator=square  SaturateOnIntegerOverflow=on
  Subtract : Sum  Inputs=+-
  Subtract1 : Sum  Inputs=+-
  Propellent_inertia : Outport
  wires:
  X_cg_oxi_engine/1 -> Square/1
  Square3/1 -> Subtract1/1, Subtract/1
  Square/1 -> Subtract/2
  mass_oxi/1 -> Multiply/2
  Subtract/1 -> Multiply/1
  Oxi_inertia/1 -> Add/1
  X_cg_fuel_engine/1 -> Square2/1
  Square2/1 -> Subtract1/2
  Subtract1/1 -> Multiply1/1
  mass_fuel/1 -> Multiply1/2
  Fuel_inertia/1 -> Add1/2
  Constant1/1 -> Create 3x3 Matrix/2
  Constant/1 -> Create 3x3 Matrix/1
  Constant3/1 -> Create 3x3 Matrix/5
  Constant5/1 -> Create 3x3 Matrix/6
  Constant7/1 -> Create 3x3 Matrix1/1
  Constant8/1 -> Create 3x3 Matrix1/2
  Constant9/1 -> Create 3x3 Matrix1/3
  Constant10/1 -> Create 3x3 Matrix1/5
  Constant11/1 -> Create 3x3 Matrix1/6
  Constant12/1 -> Create 3x3 Matrix1/7
  Constant13/1 -> Create 3x3 Matrix1/8
  Constant2/1 -> Create 3x3 Matrix/3
  Add2/1 -> Propellent_inertia/1
  Multiply1/1 -> Create 3x3 Matrix1/4, Create 3x3 Matrix1/9
  Create 3x3 Matrix1/1 -> Add1/1
  Multiply/1 -> Create 3x3 Matrix/4, Create 3x3 Matrix/9
  Constant6/1 -> Create 3x3 Matrix/8
  Constant4/1 -> Create 3x3 Matrix/7
  Create 3x3 Matrix/1 -> Add/2
  Add/1 -> Add2/1  "oxi_inertia_nose"
  Add1/1 -> Add2/2  "Fuel_inertia_nose"
  X_nose_to_engine/1 -> Add3/1
  X_cg_prop_engine/1 -> Add3/2
  Add3/1 -> Square3/1  "X_cg_prop_nose"

== system elementsLibrary/Jackalope/ascent ==
  windVelocity_E : Inport
  temperature_atm : Inport  Port=2
  pressure_atm : Inport  Port=3
  density_atm : Inport  Port=4
  thrust_B : Inport  Port=5
  motorMass : Inport  Port=6
  motorProperties : Inport  Port=7
  envConstants : Inport  Port=8
  flightState : Inport  Port=9
  towerVector : Inport  Port=10
  rocketEmptyMass : Inport  Port=11
  rocketEmptyXcg : Inport  Port=12
  motorInertias : Inport  Port=13
  kinViscosity_atm : Inport  Port=14
  airbrakeCmdAngle : Inport  Port=15
  propellantMass : Inport  Port=16
  propellantInertias : Inport  Port=17
  Ascentv1 : $bdroot/Ascentv1  ascent=ascent
  term16 : Terminator
  term17 : Terminator
  position_E : Outport
  velocity_E : Outport  Port=2
  acceleration_E : Outport  Port=3
  eulerAngles : Outport  Port=4
  angularVelocity : Outport  Port=5
  ddtQuaternions : Outport  Port=6
  quaternions : Outport  Port=7
  angularAcceleration_B : Outport  Port=8
  wires:
  windVelocity_E/1 -> Ascentv1/1
  temperature_atm/1 -> Ascentv1/2
  pressure_atm/1 -> Ascentv1/3
  density_atm/1 -> Ascentv1/4
  thrust_B/1 -> Ascentv1/5
  motorMass/1 -> Ascentv1/6
  motorProperties/1 -> Ascentv1/7
  envConstants/1 -> Ascentv1/8
  flightState/1 -> Ascentv1/9
  towerVector/1 -> Ascentv1/10
  rocketEmptyMass/1 -> Ascentv1/11
  rocketEmptyXcg/1 -> Ascentv1/12
  motorInertias/1 -> Ascentv1/13
  kinViscosity_atm/1 -> Ascentv1/14
  airbrakeCmdAngle/1 -> Ascentv1/15
  Ascentv1/1 -> position_E/1
  Ascentv1/2 -> velocity_E/1
  Ascentv1/3 -> acceleration_E/1
  Ascentv1/4 -> eulerAngles/1
  Ascentv1/5 -> angularVelocity/1
  Ascentv1/6 -> ddtQuaternions/1
  Ascentv1/7 -> quaternions/1
  Ascentv1/8 -> angularAcceleration_B/1
  propellantMass/1 -> term16/1
  propellantInertias/1 -> term17/1

== system elementsLibrary/Jackalope/avionics ==
  position_E : Inport
  orientation : Inport  Port=2
  velocity_E : Inport  Port=3
  thrust_B : Inport  Port=4
  AvionicsCharacterization : $bdroot/AvionicsCharacterization  avionics=rocket.avionics
  airbrakeCmdAngle : Outport
  descentOneDeploy : Outport  Port=2
  descentTwoDeploy : Outport  Port=3
  wires:
  position_E/1 -> AvionicsCharacterization/1
  orientation/1 -> AvionicsCharacterization/2
  velocity_E/1 -> AvionicsCharacterization/3
  thrust_B/1 -> AvionicsCharacterization/4
  AvionicsCharacterization/1 -> airbrakeCmdAngle/1
  AvionicsCharacterization/2 -> descentOneDeploy/1
  AvionicsCharacterization/3 -> descentTwoDeploy/1

== system elementsLibrary/Jackalope/environment ==
  altitude_E : Inport
  Earthv1 : $bdroot/Earthv1  environment=rocket.environment
  windVelocity_E : Outport
  Temperature : Outport  Port=2
  Pressure : Outport  Port=3
  Density : Outport  Port=4
  kinViscosity_atm : Outport  Port=5
  constants : Outport  Port=6
  wires:
  altitude_E/1 -> Earthv1/1
  Earthv1/1 -> windVelocity_E/1
  Earthv1/2 -> Temperature/1
  Earthv1/3 -> Pressure/1
  Earthv1/4 -> Density/1
  Earthv1/5 -> kinViscosity_atm/1
  Earthv1/6 -> constants/1

== system elementsLibrary/Jackalope/propulsion ==
  time : Inport
  valveCmd : Inport  Port=2
  temp_atm : Inport  Port=3
  pressure_atm : Inport  Port=4
  "density_atm " : Inport  Port=5
  SolidMotor : $bdroot/SolidMotor  propulsion=rocket.propulsion
  gnd{2..5} (4 alike) : Ground
  term{2..5} (4 alike) : Terminator
  thrust_B : Outport
  Ve_gas : Outport  Port=2
  propellantMass : Outport  Port=3
  propellantInertias : Outport  Port=4
  engineProperties : Outport  Port=5
  gasExitSpeed : Outport  Port=6
  motorMass : Outport  Port=7
  motorInertias : Outport  Port=8
  motorGeometry : Outport  Port=9
  wires:
  time/1 -> SolidMotor/1
  SolidMotor/1 -> thrust_B/1
  SolidMotor/2 -> gasExitSpeed/1
  SolidMotor/3 -> motorMass/1
  SolidMotor/4 -> motorInertias/1
  SolidMotor/5 -> motorGeometry/1
  valveCmd/1 -> term2/1
  temp_atm/1 -> term3/1
  pressure_atm/1 -> term4/1
  "density_atm "/1 -> term5/1
  gnd2/1 -> Ve_gas/1
  gnd3/1 -> propellantMass/1
  gnd4/1 -> propellantInertias/1
  gnd5/1 -> engineProperties/1

== system elementsLibrary/Jackalope/recovery ==
  windVelocity : Inport
  density_atm : Inport  Port=2
  envConstants : Inport  Port=3
  inQuaternions : Inport  Port=4
  initVelocity_E : Inport  Port=5
  initPosition_E : Inport  Port=6
  inAngVel : Inport  Port=7
  descentOneDeploy : Inport  Port=8
  descentTwoDeploy : Inport  Port=9
  flightState : Inport  Port=10
  SingleChute : $bdroot/SingleChute  recovery=rocket.recovery
  orientationP : Outport
  angularVelocityP : Outport  Port=2
  angularAccelerationP : Outport  Port=3
  angularAccelerationR : Outport  Port=4
  orientationR : Outport  Port=5
  angularVelocityR : Outport  Port=6
  posP_E : Outport  Port=7
  posR_E : Outport  Port=8
  velocityP_E : Outport  Port=9
  velocityR_E : Outport  Port=10
  accelerationR_E : Outport  Port=11
  accelerationP_E : Outport  Port=12
  wires:
  windVelocity/1 -> SingleChute/1
  density_atm/1 -> SingleChute/2
  envConstants/1 -> SingleChute/3
  inQuaternions/1 -> SingleChute/4
  initVelocity_E/1 -> SingleChute/5
  initPosition_E/1 -> SingleChute/6
  inAngVel/1 -> SingleChute/7
  descentOneDeploy/1 -> SingleChute/8
  descentTwoDeploy/1 -> SingleChute/9
  flightState/1 -> SingleChute/10
  SingleChute/1 -> orientationP/1
  SingleChute/2 -> angularVelocityP/1
  SingleChute/3 -> angularAccelerationP/1
  SingleChute/4 -> angularAccelerationR/1
  SingleChute/5 -> orientationR/1
  SingleChute/6 -> angularVelocityR/1
  SingleChute/7 -> posP_E/1
  SingleChute/8 -> posR_E/1
  SingleChute/9 -> velocityP_E/1
  SingleChute/10 -> velocityR_E/1
  SingleChute/11 -> accelerationR_E/1
  SingleChute/12 -> accelerationP_E/1

== system elementsLibrary/Jackalope/sequencer ==
  position_E : Inport
  orientation : Inport  Port=2
  velocity_E : Inport  Port=3
  thrust_B : Inport  Port=4
  descentOneDeploy : Inport  Port=5
  descentTwoDeploy : Inport  Port=6
  FSv1 : $bdroot/FSv1  sequencer=rocket.sequencer
  flightState : Outport
  towerVector : Outport  Port=2
  wires:
  position_E/1 -> FSv1/1
  orientation/1 -> FSv1/2
  velocity_E/1 -> FSv1/3
  thrust_B/1 -> FSv1/4
  descentOneDeploy/1 -> FSv1/5
  descentTwoDeploy/1 -> FSv1/6
  FSv1/1 -> flightState/1
  FSv1/2 -> towerVector/1

== system elementsLibrary/Rocktopus/ascent ==
  windVelocity_E : Inport
  temperature_atm : Inport  Port=2
  pressure_atm : Inport  Port=3
  density_atm : Inport  Port=4
  thrust_B : Inport  Port=5
  motorMass : Inport  Port=6
  motorProperties : Inport  Port=7
  envConstants : Inport  Port=8
  flightState : Inport  Port=9
  towerVector : Inport  Port=10
  rocketEmptyMass : Inport  Port=11
  rocketEmptyXcg : Inport  Port=12
  motorInertias : Inport  Port=13
  kinViscosity_atm : Inport  Port=14
  airbrakeCmdAngle : Inport  Port=15
  propellantMass : Inport  Port=16
  propellantInertias : Inport  Port=17
  Ascentv2 : $bdroot/Ascentv2  ascent=rocket.ascent
  term13 : Terminator
  term6 : Terminator
  position_E : Outport
  velocity_E : Outport  Port=2
  acceleration_E : Outport  Port=3
  eulerAngles : Outport  Port=4
  angularVelocity : Outport  Port=5
  ddtQuaternions : Outport  Port=6
  quaternions : Outport  Port=7
  angularAcceleration_B : Outport  Port=8
  wires:
  windVelocity_E/1 -> Ascentv2/1
  temperature_atm/1 -> Ascentv2/2
  pressure_atm/1 -> Ascentv2/3
  density_atm/1 -> Ascentv2/4
  thrust_B/1 -> Ascentv2/5
  propellantMass/1 -> Ascentv2/6
  motorProperties/1 -> Ascentv2/7
  envConstants/1 -> Ascentv2/8
  flightState/1 -> Ascentv2/9
  towerVector/1 -> Ascentv2/10
  rocketEmptyMass/1 -> Ascentv2/11
  rocketEmptyXcg/1 -> Ascentv2/12
  propellantInertias/1 -> Ascentv2/13
  kinViscosity_atm/1 -> Ascentv2/14
  airbrakeCmdAngle/1 -> Ascentv2/15
  Ascentv2/1 -> position_E/1
  Ascentv2/2 -> velocity_E/1
  Ascentv2/3 -> acceleration_E/1
  Ascentv2/4 -> eulerAngles/1
  Ascentv2/5 -> angularVelocity/1
  Ascentv2/6 -> ddtQuaternions/1
  Ascentv2/7 -> quaternions/1
  Ascentv2/8 -> angularAcceleration_B/1
  motorMass/1 -> term6/1
  motorInertias/1 -> term13/1

== system elementsLibrary/Rocktopus/avionics ==
  position_E : Inport
  orientation : Inport  Port=2
  velocity_E : Inport  Port=3
  thrust_B : Inport  Port=4
  AvionicsCharacterization : $bdroot/AvionicsCharacterization  avionics=rocket.avionics
  airbrakeCmdAngle : Outport
  descentOneDeploy : Outport  Port=2
  descentTwoDeploy : Outport  Port=3
  wires:
  position_E/1 -> AvionicsCharacterization/1
  orientation/1 -> AvionicsCharacterization/2
  velocity_E/1 -> AvionicsCharacterization/3
  thrust_B/1 -> AvionicsCharacterization/4
  AvionicsCharacterization/1 -> airbrakeCmdAngle/1
  AvionicsCharacterization/2 -> descentOneDeploy/1
  AvionicsCharacterization/3 -> descentTwoDeploy/1

== system elementsLibrary/Rocktopus/environment ==
  altitude_E : Inport
  Earthv1 : $bdroot/Earthv1  environment=rocket.environment
  windVelocity_E : Outport
  Temperature : Outport  Port=2
  Pressure : Outport  Port=3
  Density : Outport  Port=4
  kinViscosity_atm : Outport  Port=5
  constants : Outport  Port=6
  wires:
  altitude_E/1 -> Earthv1/1
  Earthv1/1 -> windVelocity_E/1
  Earthv1/2 -> Temperature/1
  Earthv1/3 -> Pressure/1
  Earthv1/4 -> Density/1
  Earthv1/5 -> kinViscosity_atm/1
  Earthv1/6 -> constants/1
